simulink model "mex_sfunction_simulink"  (R2024a)
settings: Solver=ode4  StartTime=0.0  StopTime=0.015  FixedStep=5e-6  RelTol=1e-3
settings Model: Creator=scut_  LastModifiedBy=Heisenberg
settings RTWCC: GPUComputeCapability=3.5

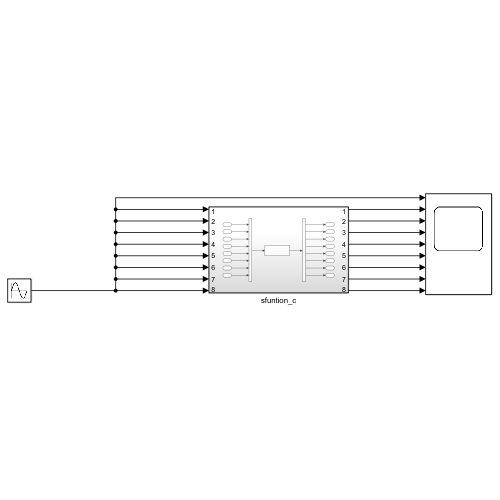
[thumbnail: Simulink's stored preview of the top-level diagram]
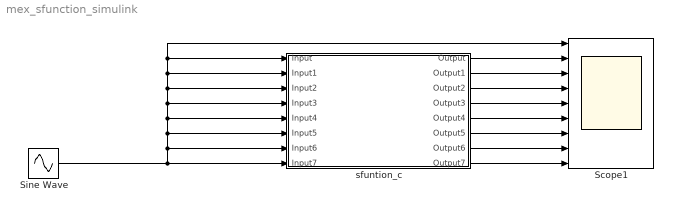
== system mex_sfunction_simulink ==
  Scope1 : Scope  NumInputPorts=9
  Sine Wave : Sin  Frequency=100*2*pi  SampleTime=0
  sfuntion_c : Subsystem
  wires:
  sfuntion_c/1(Output) -> Scope1/2
  Sine Wave/1 -> sfuntion_c/1(Input), Scope1/1, sfuntion_c/2(Input1), sfuntion_c/3(Input2), sfuntion_c/4(Input3), sfuntion_c/5(Input4), sfuntion_c/6(Input5), sfuntion_c/7(Input6), sfuntion_c/8(Input7)
  sfuntion_c/2(Output1) -> Scope1/3
  sfuntion_c/3(Output2) -> Scope1/4
  sfuntion_c/4(Output3) -> Scope1/5
  sfuntion_c/5(Output4) -> Scope1/6
  sfuntion_c/6(Output5) -> Scope1/7
  sfuntion_c/7(Output6) -> Scope1/8
  sfuntion_c/8(Output7) -> Scope1/9

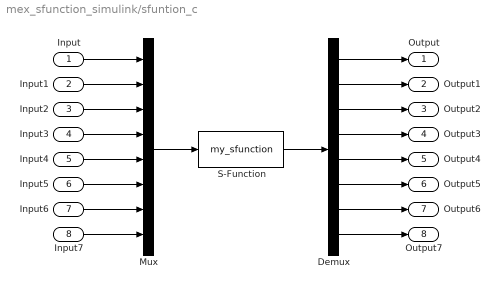
== system mex_sfunction_simulink/sfuntion_c ==
  Input : Inport
  Input1 : Inport  Port=2
  Input2 : Inport  Port=3
  Input3 : Inport  Port=4
  Input4 : Inport  Port=5
  Input5 : Inport  Port=6
  Input6 : Inport  Port=7
  Input7 : Inport  Port=8
  Demux : Demux  Outputs=8
  Mux : Mux  Inputs=8
  S-Function : S-Function  FunctionName=my_sfunction  SFunctionDeploymentMode=off  EnableBusSupport=off
  Output : Outport
  Output1 : Outport  Port=2
  Output2 : Outport  Port=3
  Output3 : Outport  Port=4
  Output4 : Outport  Port=5
  Output5 : Outport  Port=6
  Output6 : Outport  Port=7
  Output7 : Outport  Port=8
  wires:
  Input/1 -> Mux/1
  Demux/1 -> Output/1
  S-Function/1 -> Demux/1
  Mux/1 -> S-Function/1
  Input1/1 -> Mux/2
  Demux/2 -> Output1/1
  Input2/1 -> Mux/3
  Input3/1 -> Mux/4
  Input4/1 -> Mux/5
  Demux/3 -> Output2/1
  Demux/4 -> Output3/1
  Demux/5 -> Output4/1
  Input6/1 -> Mux/7
  Input5/1 -> Mux/6
  Input7/1 -> Mux/8
  Demux/8 -> Output7/1
  Demux/7 -> Output6/1
  Demux/6 -> Output5/1
